simulink subsystem "Baseline"  (R2020b)
settings: Solver=VariableStepAuto  StartTime=0.0  StopTime=10.0  RelTol=1e-3
undefined symbols (not defined in the file): Baseline, ControllersLib, SimIn
libraries: ComponentsLib x13, AdaptiveLib x1, libAxisTransformations x1
settings Model: Creator=tbritton  LastModifiedBy=azmol

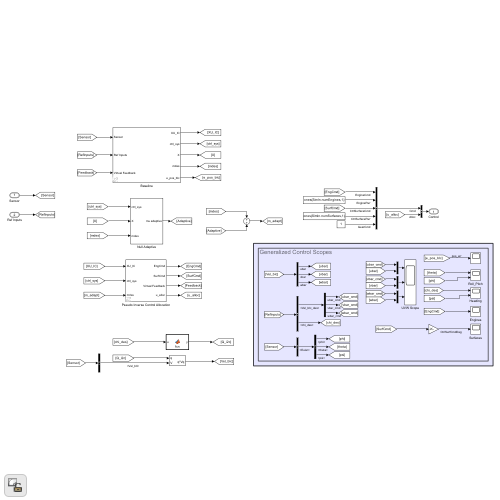
[thumbnail: Simulink's stored preview of the top-level diagram]
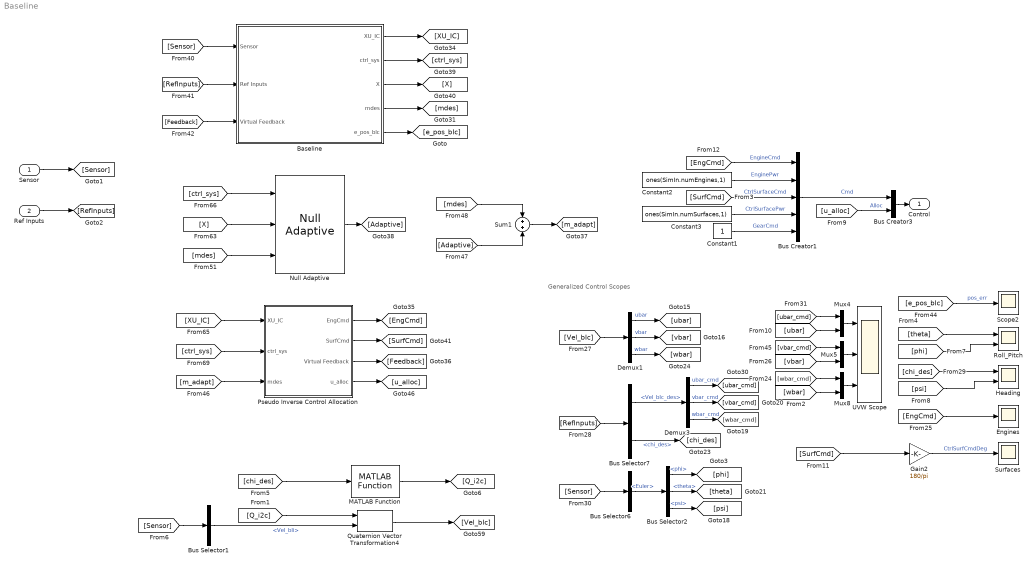
== system Baseline ==
  note: Generalized Control Scopes
  Sensor : Inport  OutDataTypeStr=Bus: SensorBus
  Ref Inputs : Inport  Port=2  OutDataTypeStr=Bus: BUS_REF_INPUT
  Baseline : Subsystem  AncestorBlock=ControllersLib/Baseline
  Bus Creator1 : BusCreator  Inputs=5  OutDataTypeStr=Bus: BUS_CMD
  Bus Creator3 : BusCreator  Inputs=2
  Bus Selector1 : BusSelector  OutputSignals=Vel_bIi
  Bus Selector2 : BusSelector  OutputSignals=phi,theta,psi
  Bus Selector6 : BusSelector  OutputSignals=Euler
  Bus Selector7 : BusSelector  OutputSignals=Vel_bIc_des,chi_des
  Constant1 : Constant
  Constant2 : Constant  Value=ones(SimIn.numEngines,1)
  Constant3 : Constant  Value=ones(SimIn.numSurfaces,1)
  Demux1 : Demux  Outputs=3
  Demux3 : Demux  Outputs=3
  Engines : Scope
  Gain2 : Gain  Gain=180/pi
  Heading : Scope  NumInputPorts=2
  MATLAB Function : ComponentsLib/ConvertToControlFrame/MATLAB Function  SystemSampleTime=-1  VariantActivationTime=update diagram  Latency=0  AutoFrameSizeCalculation=off
  Mux4 : Mux  Inputs=2
  Mux5 : Mux  Inputs=2
  Mux8 : Mux  Inputs=2
  Null Adaptive : AdaptiveLib/Null Adaptive  SystemSampleTime=-1  VariantActivationTime=update diagram  Latency=0  AutoFrameSizeCalculation=off
  Pseudo Inverse Control Allocation : Subsystem  AncestorBlock=AllocatorsLib/Pseudo Inverse Control Allocation
  Quaternion Vector Transformation4 : libAxisTransformations/Quaternion Vector Transformation  n=0
  Roll_Pitch : Scope  NumInputPorts=2
  Scope2 : Scope
  Sum1 : Sum
  Surfaces : Scope
  UVW Scope : Scope  NumInputPorts=3
  Control : Outport  OutDataTypeStr=Bus: BUS_CONTROL  VectorParamsAs1DForOutWhenUnconnected=off
  wires:
  Ref Inputs/1 -> [RefInputs]
  [u_alloc] -> Bus Creator3/2  "Alloc"
  Bus Creator3/1 -> Control/1
  Constant1/1 -> Bus Creator1/5  "GearCmd"
  [SurfCmd] -> Bus Creator1/3  "CtrlSurfaceCmd"
  Bus Creator1/1 -> Bus Creator3/1  "Cmd"
  Sensor/1 -> [Sensor]
  [EngCmd] -> Bus Creator1/1  "EngineCmd"
  Constant2/1 -> Bus Creator1/2  "EnginePwr"
  Constant3/1 -> Bus Creator1/4  "CtrlSurfacePwr"
  [Sensor] -> Baseline/1(Sensor)
  [RefInputs] -> Baseline/2(Ref Inputs)
  [Feedback] -> Baseline/3(Virtual Feedback)
  Baseline/4(mdes) -> [mdes]
  [m_adapt] -> Pseudo Inverse Control Allocation/3(mdes)
  Pseudo Inverse Control Allocation/3(Virtual Feedback) -> [Feedback]
  Baseline/1(XU_IC) -> [XU_IC]
  Pseudo Inverse Control Allocation/1(EngCmd) -> [EngCmd]
  [ctrl_sys] -> Null Adaptive/1
  [mdes] -> Null Adaptive/3
  [X] -> Null Adaptive/2
  Null Adaptive/1 -> [Adaptive]
  Baseline/2(ctrl_sys) -> [ctrl_sys]
  Baseline/3(X) -> [X]
  Sum1/1 -> [m_adapt]
  [mdes] -> Sum1/1
  [Adaptive] -> Sum1/2
  Pseudo Inverse Control Allocation/2(SurfCmd) -> [SurfCmd]
  Pseudo Inverse Control Allocation/4(u_alloc) -> [u_alloc]
  [XU_IC] -> Pseudo Inverse Control Allocation/1(XU_IC)
  [ctrl_sys] -> Pseudo Inverse Control Allocation/2(ctrl_sys)
  Bus Selector1/1 -> Quaternion Vector Transformation4/2  "<Vel_bIi>"
  [Q_i2c] -> Quaternion Vector Transformation4/1
  [chi_des] -> MATLAB Function/1
  Quaternion Vector Transformation4/1 -> [Vel_bIc]
  MATLAB Function/1 -> [Q_i2c]
  [Sensor] -> Bus Selector1/1
  Demux1/3 -> [wbar]  "wbar"
  [wbar_cmd] -> Mux8/1
  Bus Selector7/2 -> [chi_des]  "<chi_des>"
  [Vel_bIc] -> Demux1/1
  Demux3/1 -> [ubar_cmd]  "ubar_cmd"
  Bus Selector7/1 -> Demux3/1  "<Vel_bIc_des>"
  [EngCmd] -> Engines/1
  Demux1/2 -> [vbar]  "vbar"
  [psi] -> Heading/2
  Bus Selector2/2 -> [theta]  "<theta>"
  [theta] -> Roll_Pitch/1
  Gain2/1 -> Surfaces/1  "CtrlSurfCmdDeg"
  Bus Selector2/3 -> [psi]  "<psi>"
  Mux8/1 -> UVW Scope/3
  Bus Selector2/1 -> [phi]  "<phi>"
  Bus Selector6/1 -> Bus Selector2/1  "<Euler>"
  [e_pos_bIc] -> Scope2/1  "pos_err"
  Demux3/2 -> [vbar_cmd]  "vbar_cmd"
  [phi] -> Roll_Pitch/2
  [wbar] -> Mux8/2
  [RefInputs] -> Bus Selector7/1
  [Sensor] -> Bus Selector6/1
  [ubar] -> Mux4/2
  [chi_des] -> Heading/1
  [SurfCmd] -> Gain2/1
  [vbar] -> Mux5/2
  [ubar_cmd] -> Mux4/1
  [vbar_cmd] -> Mux5/1
  Mux5/1 -> UVW Scope/2
  Demux3/3 -> [wbar_cmd]  "wbar_cmd"
  Mux4/1 -> UVW Scope/1
  Demux1/1 -> [ubar]  "ubar"
  Baseline/5(e_pos_blc) -> [e_pos_bIc]

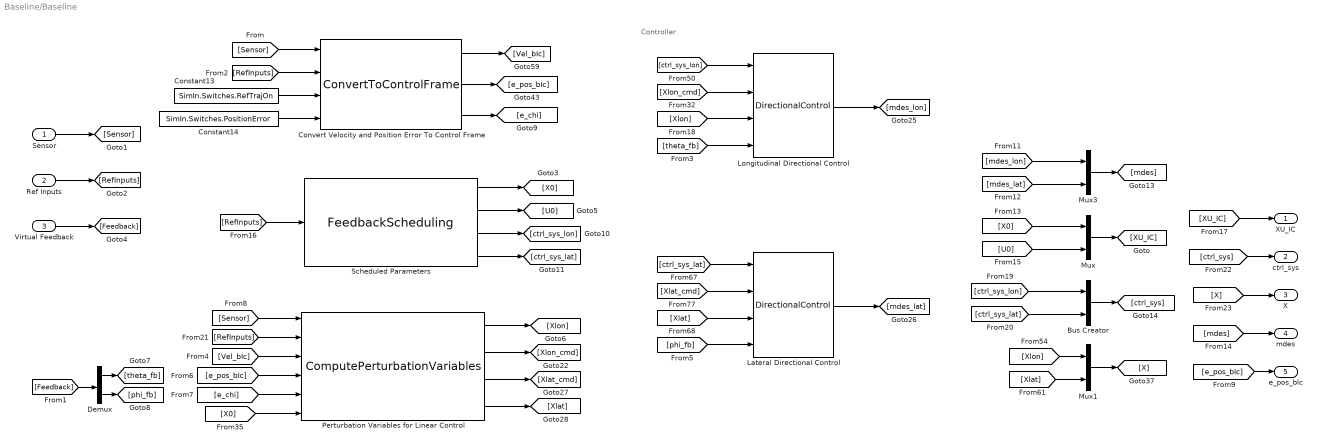
== system Baseline/Baseline ==
  note: Controller
  Sensor : Inport  OutDataTypeStr=Bus: SensorBus
  Ref Inputs : Inport  Port=2  OutDataTypeStr=Bus: BUS_REF_INPUT
  Virtual Feedback : Inport  Port=3
  Bus Creator : BusCreator  Inputs=2
  Constant13 : Constant  Value=SimIn.Switches.RefTrajOn
  Constant14 : Constant  Value=SimIn.Switches.PositionError
  Convert Velocity and Position Error To Control Frame : ComponentsLib/ConvertToControlFrame  SystemSampleTime=-1  VariantActivationTime=update diagram  Latency=0  AutoFrameSizeCalculation=off
  Demux : Demux  Outputs=2
  Lateral Directional Control : ComponentsLib/DirectionalControl  SystemSampleTime=-1  VariantActivationTime=update diagram  Latency=0  AutoFrameSizeCalculation=off
  Longitudinal Directional Control : ComponentsLib/DirectionalControl  SystemSampleTime=-1  VariantActivationTime=update diagram  Latency=0  AutoFrameSizeCalculation=off
  Mux : Mux  Inputs=2
  Mux1 : Mux  Inputs=2
  Mux3 : Mux  Inputs=2
  Perturbation Variables for Linear Control : ComponentsLib/ComputePerturbationVariables  SystemSampleTime=-1  VariantActivationTime=update diagram  Latency=0  AutoFrameSizeCalculation=off
  Scheduled Parameters : ComponentsLib/FeedbackScheduling  SystemSampleTime=-1  VariantActivationTime=update diagram  Latency=0  AutoFrameSizeCalculation=off
  XU_IC : Outport
  ctrl_sys : Outport  Port=2
  X : Outport  Port=3
  mdes : Outport  Port=4
  e_pos_blc : Outport  Port=5
  wires:
  [e_pos_bIc] -> e_pos_blc/1
  [X0] -> Perturbation Variables for Linear Control/6
  Perturbation Variables for Linear Control/1 -> [Xlon]
  [Sensor] -> Perturbation Variables for Linear Control/1
  Perturbation Variables for Linear Control/3 -> [Xlat_cmd]
  Sensor/1 -> [Sensor]
  Scheduled Parameters/1 -> [X0]
  Ref Inputs/1 -> [RefInputs]
  [RefInputs] -> Convert Velocity and Position Error To Control Frame/2
  Convert Velocity and Position Error To Control Frame/1 -> [Vel_bIc]
  Convert Velocity and Position Error To Control Frame/2 -> [e_pos_bIc]
  Scheduled Parameters/3 -> [ctrl_sys_lon]
  [e_pos_bIc] -> Perturbation Variables for Linear Control/4
  Perturbation Variables for Linear Control/4 -> [Xlat]
  [RefInputs] -> Scheduled Parameters/1
  Perturbation Variables for Linear Control/2 -> [Xlon_cmd]
  Convert Velocity and Position Error To Control Frame/3 -> [e_chi]
  [Sensor] -> Convert Velocity and Position Error To Control Frame/1
  [Vel_bIc] -> Perturbation Variables for Linear Control/3
  Constant13/1 -> Convert Velocity and Position Error To Control Frame/3
  [RefInputs] -> Perturbation Variables for Linear Control/2
  Constant14/1 -> Convert Velocity and Position Error To Control Frame/4
  [e_chi] -> Perturbation Variables for Linear Control/5
  Scheduled Parameters/2 -> [U0]
  Scheduled Parameters/4 -> [ctrl_sys_lat]
  [Xlon_cmd] -> Longitudinal Directional Control/2
  Lateral Directional Control/1 -> [mdes_lat]
  [ctrl_sys_lat] -> Lateral Directional Control/1
  [ctrl_sys_lon] -> Longitudinal Directional Control/1
  Longitudinal Directional Control/1 -> [mdes_lon]
  [Xlat] -> Lateral Directional Control/3
  [Xlon] -> Longitudinal Directional Control/3
  [Xlat_cmd] -> Lateral Directional Control/2
  Virtual Feedback/1 -> [Feedback]
  [Feedback] -> Demux/1
  Demux/2 -> [phi_fb]
  Demux/1 -> [theta_fb]
  [theta_fb] -> Longitudinal Directional Control/4
  [phi_fb] -> Lateral Directional Control/4
  [mdes_lon] -> Mux3/1
  [mdes_lat] -> Mux3/2
  Mux3/1 -> [mdes]
  [mdes] -> mdes/1
  [X0] -> Mux/1
  [U0] -> Mux/2
  Mux/1 -> [XU_IC]
  [XU_IC] -> XU_IC/1
  [ctrl_sys_lon] -> Bus Creator/1
  [ctrl_sys_lat] -> Bus Creator/2
  Bus Creator/1 -> [ctrl_sys]
  [ctrl_sys] -> ctrl_sys/1
  Mux1/1 -> [X]
  [Xlon] -> Mux1/1
  [Xlat] -> Mux1/2
  [X] -> X/1

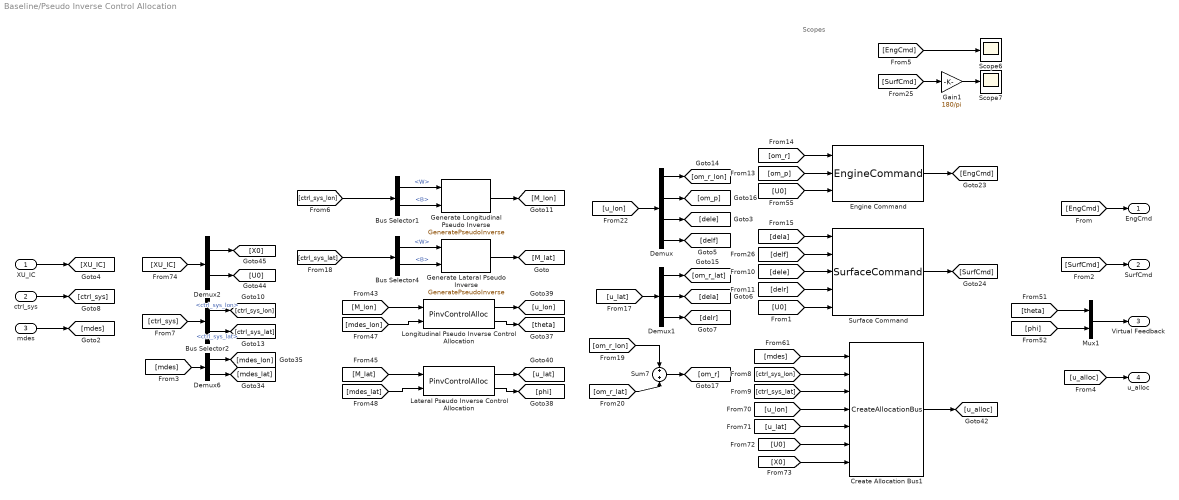
== system Baseline/Pseudo Inverse Control Allocation ==
  note: Scopes
  XU_IC : Inport
  ctrl_sys : Inport  Port=2
  mdes : Inport  Port=3
  Bus Selector1 : BusSelector  OutputSignals=W,B
  Bus Selector2 : BusSelector  OutputSignals=ctrl_sys_lon,ctrl_sys_lat
  Bus Selector4 : BusSelector  OutputSignals=W,B
  Create Allocation Bus1 : ComponentsLib/CreateAllocationBus  SystemSampleTime=-1  VariantActivationTime=update diagram  Latency=0  AutoFrameSizeCalculation=off
  Demux : Demux  Outputs=[8 1 1 1]
  Demux1 : Demux  Outputs=[8 1 1]
  Demux2 : Demux  Outputs=[12 13]
  Demux6 : Demux  Outputs=[3 3]
  Engine Command : ComponentsLib/EngineCommand  SystemSampleTime=-1  VariantActivationTime=update diagram  Latency=0  AutoFrameSizeCalculation=off
  Gain1 : Gain  Gain=180/pi
  Generate Lateral Pseudo Inverse : ComponentsLib/GeneratePseudoInverse  SystemSampleTime=-1  VariantActivationTime=update diagram  Latency=0  AutoFrameSizeCalculation=off
  Generate Longitudinal Pseudo Inverse : ComponentsLib/GeneratePseudoInverse  SystemSampleTime=-1  VariantActivationTime=update diagram  Latency=0  AutoFrameSizeCalculation=off
  Lateral Pseudo Inverse Control Allocation : ComponentsLib/PinvControlAlloc  SystemSampleTime=-1  VariantActivationTime=update diagram  Latency=0  AutoFrameSizeCalculation=off
  Longitudinal Pseudo Inverse Control Allocation : ComponentsLib/PinvControlAlloc  SystemSampleTime=-1  VariantActivationTime=update diagram  Latency=0  AutoFrameSizeCalculation=off
  Mux1 : Mux  Inputs=2
  Scope6 : Scope
  Scope7 : Scope
  Sum7 : Sum
  Surface Command : ComponentsLib/SurfaceCommand  SystemSampleTime=-1  VariantActivationTime=update diagram  Latency=0  AutoFrameSizeCalculation=off
  EngCmd : Outport
  SurfCmd : Outport  Port=2
  Virtual Feedback : Outport  Port=3
  u_alloc : Outport  Port=4
  wires:
  Lateral Pseudo Inverse Control Allocation/2 -> [phi]
  Longitudinal Pseudo Inverse Control Allocation/1 -> [u_lon]
  [theta] -> Mux1/1
  [mdes_lat] -> Lateral Pseudo Inverse Control Allocation/2
  [phi] -> Mux1/2
  [mdes_lon] -> Longitudinal Pseudo Inverse Control Allocation/2
  Lateral Pseudo Inverse Control Allocation/1 -> [u_lat]
  Longitudinal Pseudo Inverse Control Allocation/2 -> [theta]
  Mux1/1 -> Virtual Feedback/1
  [M_lon] -> Longitudinal Pseudo Inverse Control Allocation/1
  [M_lat] -> Lateral Pseudo Inverse Control Allocation/1
  Demux/3 -> [dele]
  Demux/2 -> [om_p]
  [u_lat] -> Demux1/1
  [om_r_lat] -> Sum7/2
  [om_r_lon] -> Sum7/1
  Sum7/1 -> [om_r]
  [u_lon] -> Demux/1
  Demux1/2 -> [dela]
  Demux1/1 -> [om_r_lat]
  Demux/1 -> [om_r_lon]
  Demux/4 -> [delf]
  Demux1/3 -> [delr]
  Engine Command/1 -> [EngCmd]
  Surface Command/1 -> [SurfCmd]
  [U0] -> Engine Command/3
  [dele] -> Surface Command/3
  [delf] -> Surface Command/2
  [delr] -> Surface Command/4
  [om_p] -> Engine Command/2
  [om_r] -> Engine Command/1
  [U0] -> Surface Command/5
  [dela] -> Surface Command/1
  [EngCmd] -> EngCmd/1
  [SurfCmd] -> SurfCmd/1
  Demux2/2 -> [U0]
  [U0] -> Create Allocation Bus1/6
  [u_lon] -> Create Allocation Bus1/4
  Create Allocation Bus1/1 -> [u_alloc]
  [u_lat] -> Create Allocation Bus1/5
  [XU_IC] -> Demux2/1
  [X0] -> Create Allocation Bus1/7
  Demux2/1 -> [X0]
  [mdes] -> Create Allocation Bus1/1
  Demux6/2 -> [mdes_lat]
  Demux6/1 -> [mdes_lon]
  [mdes] -> Demux6/1
  mdes/1 -> [mdes]
  XU_IC/1 -> [XU_IC]
  ctrl_sys/1 -> [ctrl_sys]
  [u_alloc] -> u_alloc/1
  Gain1/1 -> Scope7/1
  [SurfCmd] -> Gain1/1
  [EngCmd] -> Scope6/1
  [ctrl_sys_lat] -> Bus Selector4/1
  Bus Selector1/1 -> Generate Longitudinal Pseudo Inverse/1  "<W>"
  [ctrl_sys_lon] -> Bus Selector1/1
  Generate Longitudinal Pseudo Inverse/1 -> [M_lon]
  Bus Selector4/1 -> Generate Lateral Pseudo Inverse/1  "<W>"
  Generate Lateral Pseudo Inverse/1 -> [M_lat]
  Bus Selector4/2 -> Generate Lateral Pseudo Inverse/2  "<B>"
  Bus Selector1/2 -> Generate Longitudinal Pseudo Inverse/2  "<B>"
  [ctrl_sys] -> Bus Selector2/1
  Bus Selector2/1 -> [ctrl_sys_lon]  "<ctrl_sys_lon>"
  Bus Selector2/2 -> [ctrl_sys_lat]  "<ctrl_sys_lat>"
  [ctrl_sys_lon] -> Create Allocation Bus1/2
  [ctrl_sys_lat] -> Create Allocation Bus1/3
